simulink model "test"  (R2018b)
settings: Solver=VariableStepAuto  StartTime=0.0  StopTime=10.0  RelTol=1e-3
values from neighbouring files (symbols this model uses):
  A_bike = [0 g/h_real ; 1 0]    [configuration.m]
  A_bike_dis_prediction = A_bike_dis^d_delay    [configuration.m]    (also in prediction_smith.m)
  B_bike = [1 ; 0]    [configuration.m]
  B_bike_dis_prediction = vec_powers_AB    [configuration.m]    (also in prediction_smith.m)
  C1_bike = a_real/(b_real*h_real)    (= 0.392543973584)    [configuration.m]
  C2_bike = 1/(b_real*h_real)    (= 1.15454109878)    [configuration.m]
  C_ini = [C1_bike*input_velocity C2_bike*input_velocity^2]    [configuration.m]
  D = zeros(3,1)    [configuration_pidTuning.m]
  d_delay = delay_tf_steering/Ts    (= 0)    [configuration.m]    (also in prediction_smith.m = 3)
  D_steering_position = 0.0    (= 0)    [configuration.m]
  delay_tf_steering = 0    [configuration.m]
  den_tf_steering = [1 245.9 0]    [configuration.m]
  den_tf_steering_dis = [den_tf_steering_dis 0] - [0 den_tf_steering_dis]    [configuration.m]
  I_steering_position = 1    [configuration.m]    (also in simulate_bike.m = 30)
  initial_states = [deg2rad(-2) deg2rad(0) deg2rad(0)]    [configuration.m]    (also in configuration_pidTuning.m)
  input_velocity = 4    [configuration.m]    (also in configuration_pidTuning.m = 3)
  K_feedforward_steering = 0    [configuration.m]
  K_fullbike = 1    [configuration.m]
  lqr_gains = zeros(length(velocity_lqr),1+size(A_bike,1))    [lqr_design.m]
  max_steering_motor_speed = 0.9    [configuration.m]    (also in configuration_pidTuning.m = 7.5)
  min_steering_motor_speed = -0.9    [configuration.m]    (also in configuration_pidTuning.m = -7.5)
  num_tf_steering = [253.4]    [configuration.m]
  num_tf_steering_dis = [num_tf_steering_dis 0]    [configuration.m]
  P_steering_position = 10    [configuration.m]    (also in simulate_bike.m = 30)
  smith_fullbike = 1    [configuration.m]
  smith_steering = 0    [configuration.m]
  Ts = 0.01    [configuration.m]    (also in configuration_pidTuning.m = 0.04)
  velocity_lqr = [input_velocity - 0.1 , input_velocity , input_velocity + 0.1]    [lqr_design.m]
undefined symbols (not defined in the file or in its folder): a_steering_filter, b_steering_filter
libraries: simulink x3
settings Model: Creator=maximef  LastModifiedBy=maximef

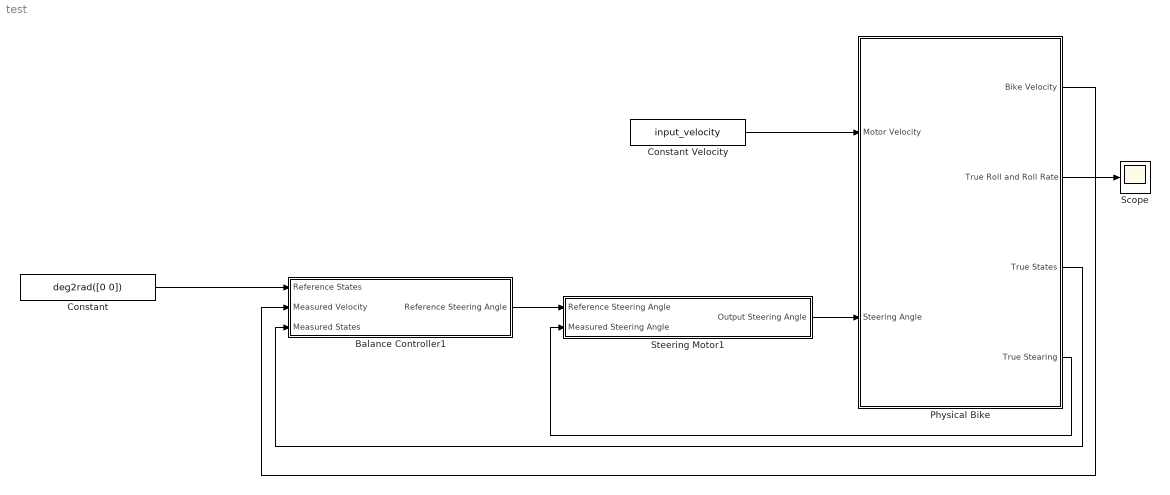
== system test ==
  Balance Controller1 : Subsystem  SystemSampleTime=Ts
  Constant : Constant  Value=deg2rad([0 0])
  Constant Velocity : Constant  Value=input_velocity
  Physical Bike : Subsystem
  Scope : Scope
  Steering Motor1 : Subsystem
  wires:
  Balance Controller1/1(Reference Steering Angle) -> Steering Motor1/1(Reference Steering Angle)
  Steering Motor1/1(Output Steering Angle) -> Physical Bike/2(Steering Angle)
  Physical Bike/3(True States) -> Balance Controller1/3(Measured States)
  Physical Bike/1(Bike Velocity) -> Balance Controller1/2(Measured Velocity)
  Physical Bike/2(True Roll and Roll Rate) -> Scope/1
  Physical Bike/4(True Stearing) -> Steering Motor1/2(Measured Steering Angle)
  Constant Velocity/1 -> Physical Bike/1(Motor Velocity)
  Constant/1 -> Balance Controller1/1(Reference States)

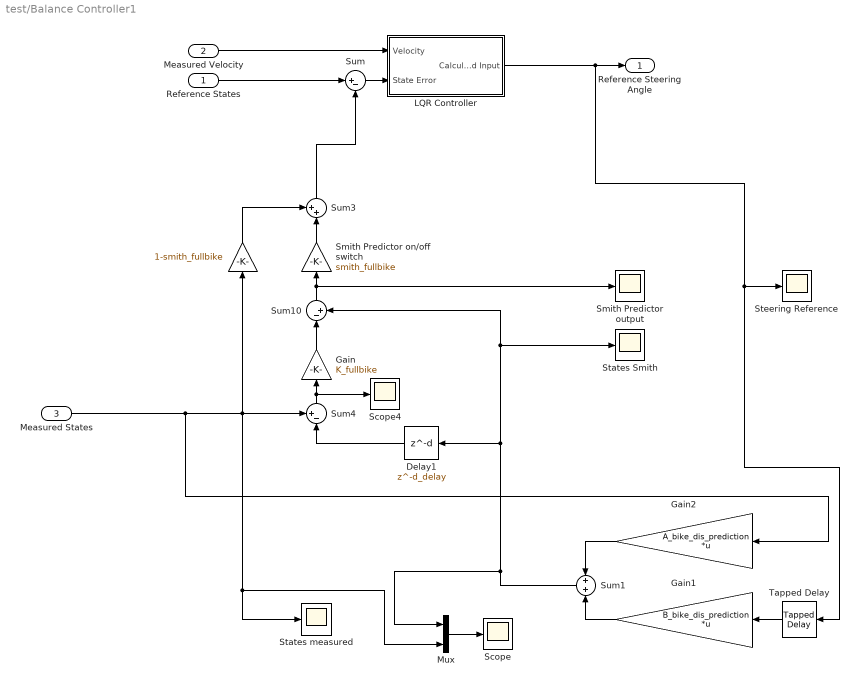
== system test/Balance Controller1 ==
  Reference States : Inport
  Measured Velocity : Inport  Port=2
  Measured States : Inport  Port=3
  " " : Gain  Gain=1-smith_fullbike
  Delay1 : Delay  DelayLength=d_delay  SampleTime=Ts
  Gain : Gain  Gain=K_fullbike
  Gain1 : Gain  Gain=B_bike_dis_prediction  Multiplication=Matrix(K*u)
  Gain2 : Gain  Gain=A_bike_dis_prediction  Multiplication=Matrix(K*u)
  LQR Controller : Subsystem  TreatAsAtomicUnit=on  SystemSampleTime=Ts
  Mux : Mux  Inputs=2
  Scope : Scope
  Scope4 : Scope
  Smith Predictor on/off switch : Gain  Gain=smith_fullbike
  Smith Predictor output : Scope
  States Smith : Scope
  States measured : Scope
  Steering Reference : Scope
  Sum : Sum  Inputs=|+-
  Sum1 : Sum
  Sum10 : Sum  Inputs=|-+
  Sum3 : Sum  Inputs=++|
  Sum4 : Sum  Inputs=+-|
  Tapped Delay : simulink/Discrete/Tapped Delay  vinit=0.0  samptime=Ts  NumDelays=d_delay  DelayOrder=Oldest  includeCurrent=off
  Reference Steering Angle : Outport
  wires:
  Sum/1 -> LQR Controller/2(State Error)
  " "/1 -> Sum3/1
  Sum3/1 -> Sum/2
  Gain/1 -> Sum10/1
  Delay1/1 -> Sum4/2
  Smith Predictor on/off switch/1 -> Sum3/2
  Sum10/1 -> Smith Predictor output/1, Smith Predictor on/off switch/1
  Sum4/1 -> Scope4/1, Gain/1
  LQR Controller/1(Calculated Input) -> Tapped Delay/1, Steering Reference/1, Reference Steering Angle/1
  Measured Velocity/1 -> LQR Controller/1(Velocity)
  Gain1/1 -> Sum1/2
  Tapped Delay/1 -> Gain1/1
  Gain2/1 -> Sum1/1
  Sum1/1 -> Sum10/2, States Smith/1, Delay1/1, Mux/1
  Mux/1 -> Scope/1
  Measured States/1 -> Gain2/1, " "/1, States measured/1, Mux/2, Sum4/1
  Reference States/1 -> Sum/1

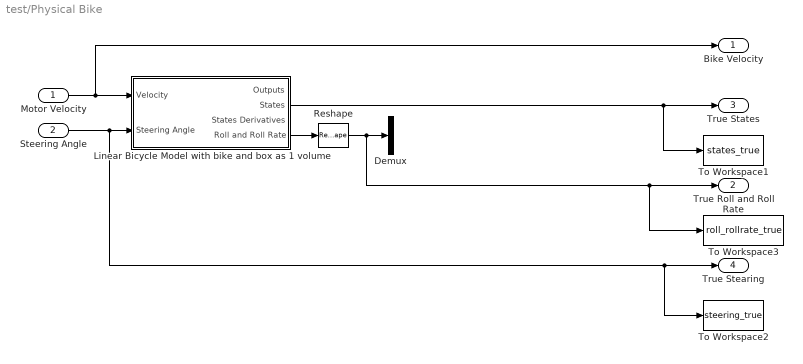
== system test/Physical Bike ==
  Motor Velocity : Inport
  Steering Angle : Inport  Port=2
  Demux : Demux  Outputs=2
  Linear Bicycle Model with bike and box as 1 volume : Subsystem
  Reshape : Reshape
  To Workspace1 : ToWorkspace  VariableName=states_true  SaveFormat=Timeseries  SampleTime=-1
  To Workspace2 : ToWorkspace  VariableName=steering_true  SaveFormat=Timeseries  SampleTime=-1
  To Workspace3 : ToWorkspace  VariableName=roll_rollrate_true  SaveFormat=Timeseries  SampleTime=-1
  Bike Velocity : Outport
  True Roll and Roll Rate : Outport  Port=2
  True States : Outport  Port=3
  True Stearing : Outport  Port=4
  wires:
  Steering Angle/1 -> To Workspace2/1, True Stearing/1, Linear Bicycle Model with bike and box as 1 volume/2(Steering Angle)
  Motor Velocity/1 -> Bike Velocity/1, Linear Bicycle Model with bike and box as 1 volume/1(Velocity)
  Linear Bicycle Model with bike and box as 1 volume/2(States) -> To Workspace1/1, True States/1
  Linear Bicycle Model with bike and box as 1 volume/4(Roll and Roll Rate) -> Reshape/1
  Reshape/1 -> To Workspace3/1, True Roll and Roll Rate/1, Demux/1

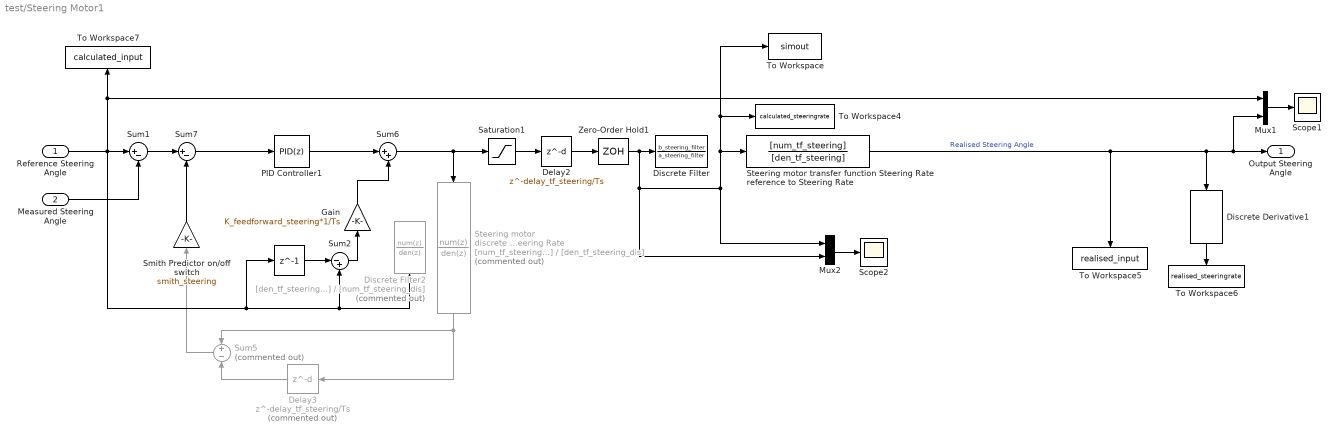
== system test/Steering Motor1 ==
  Reference Steering Angle : Inport
  Measured Steering Angle : Inport  Port=2
  " " : Delay  DelayLength=1  SampleTime=Ts
  Delay2 : Delay  DelayLength=delay_tf_steering/Ts  SampleTime=Ts
  Delay3 : Delay  Commented=on  DelayLength=delay_tf_steering/Ts  SampleTime=Ts
  Discrete Derivative1 : simulink/Discrete/Discrete Derivative  gainval=1.0  ICPrevScaledInput=0.0  OutMin=[]  OutMax=[]  OutDataType=fixdt(1, 16)  OutScaling=2^-10  DoSatur=off
  Discrete Filter : DiscreteFilter  Numerator=b_steering_filter  Denominator=a_steering_filter  SampleTime=Ts
  Discrete Filter2 : DiscreteFilter  Commented=on  Numerator=[den_tf_steering_dis]  Denominator=[num_tf_steering_dis]
  Gain : Gain  Gain=K_feedforward_steering*1/Ts
  Mux1 : Mux  Inputs=2
  Mux2 : Mux  Inputs=2
  PID Controller1 : simulink/Continuous/PID Controller  Controller=PID  Form=Parallel  TimeDomain=Discrete-time  SampleTime=Ts  IntegratorMethod=Forward Euler  FilterMethod=Forward Euler  ControllerParametersSource=internal  P=P_steering_position  I=I_steering_position  D=D_steering_position  UseFilter=off  N=1  TunerSelectOption=Transfer Function Based (PID Tuner App)  InitialConditionSource=internal  InitialConditionForIntegrator=0  InitialConditionForFilter=0  DifferentiatorICPrevScaledInput=0  ExternalReset=none  TrackingMode=off  Kt=1  LimitOutput=off  UpperSaturationLimit=inf  LowerSaturationLimit=-inf  LinearizeAsGain=on  AntiWindupMode=none  Kb=1  POutMin=[]  POutMax=[]  IOutMin=[]  IOutMax=[]  DOutMin=[]  DOutMax=[]  NOutMin=[]  NOutMax=[]  SumOutMin=[]  SumOutMax=[]  SaturationOutMin=[]  SaturationOutMax=[]  PParamMin=[]  PParamMax=[]  IParamMin=[]  IParamMax=[]  DParamMin=[]  DParamMax=[]  NParamMin=[]  NParamMax=[]  KbParamMin=[]  KbParamMax=[]  KtParamMin=[]  KtParamMax=[]  KbOutMin=[]  KbOutMax=[]  KtOutMin=[]  KtOutMax=[]  IntegratorOutMin=[]  IntegratorOutMax=[]  FilterOutMin=[]  FilterOutMax=[]  SumI1OutMin=[]  SumI1OutMax=[]  SumI2OutMin=[]  SumI2OutMax=[]  SumI3OutMin=[]  SumI3OutMax=[]  SumI4OutMin=[]  SumI4OutMax=[]  SumDOutMin=[]  SumDOutMax=[]  DifferentiatorOutMin=[]  DifferentiatorOutMax=[]  FilterDiffOutCoefMin=[]  FilterDiffOutCoefMax=[]  ReciprocalOutMin=[]  ReciprocalOutMax=[]  SumDenOutMin=[]  SumDenOutMax=[]  SumNumOutMin=[]  SumNumOutMax=[]  DivideOutMin=[]  DivideOutMax=[]  IntegratorContinuousStateAttributes=''  IntegratorStateMustResolveToSignalObject=off  IntegratorRTWStateStorageClass=Auto  FilterContinuousStateAttributes=''  FilterStateMustResolveToSignalObject=off  FilterRTWStateStorageClass=Auto  ParallelPVariant=InternalParameters  IdealPVariant=Disabled  IVariant=InternalParameters  DVariant=InternalParameters  IntegratorVariant=Discrete  SatVariant=Disabled  AWVariant=Passthrough  PCopyVariant=Disabled  TRVariant=Disabled  FdbkBlocksVariant=Forward  IdealPFdbkVariant=Disabled  SatFdbkVariant=Disabled  DerivativeFilterVariant=Differentiator  NVariant=Passthrough  NCopyVariant=Disabled_SignalSpec  FilterICVariant=InternalICsDifferentiator  IntegratorICVariant=InternalICs  ExternalResetVariant=Disabled  TRSumVariant=Passthrough  SumFdbkVariant=Disabled  SumVariant=Sum_PID
  Saturation1 : Saturate  UpperLimit=max_steering_motor_speed  LowerLimit=min_steering_motor_speed
  Scope1 : Scope
  Scope2 : Scope
  Smith Predictor on/off switch : Gain  Gain=smith_steering
  Steering motor discrete transfer function Steering Rate reference to Steering Rate : DiscreteTransferFcn  Commented=on  Numerator=[num_tf_steering_dis]  Denominator=[den_tf_steering_dis]  SampleTime=Ts
  Steering motor transfer function Steering Rate reference to Steering Rate : TransferFcn  Numerator=[num_tf_steering]  Denominator=[den_tf_steering]
  Sum1 : Sum  Inputs=|+-
  Sum2 : Sum  Inputs=|-+
  Sum5 : Sum  Commented=on  Inputs=+-
  Sum6 : Sum  Inputs=|++
  Sum7 : Sum  Inputs=|+-
  To Workspace : ToWorkspace  VariableName=simout  SaveFormat=Timeseries  SampleTime=-1
  To Workspace4 : ToWorkspace  VariableName=calculated_steeringrate  SaveFormat=Timeseries  SampleTime=-1
  To Workspace5 : ToWorkspace  VariableName=realised_input  SaveFormat=Timeseries  SampleTime=-1
  To Workspace6 : ToWorkspace  VariableName=realised_steeringrate  SaveFormat=Timeseries  SampleTime=-1
  To Workspace7 : ToWorkspace  VariableName=calculated_input  SaveFormat=Timeseries  SampleTime=Ts
  Zero-Order Hold1 : ZeroOrderHold  SampleTime=Ts
  Output Steering Angle : Outport
  wires:
  Saturation1/1 -> Delay2/1
  Steering motor discrete transfer function Steering Rate reference to Steering Rate/1 -> Delay3/1, Sum5/1
  Sum5/1 -> Smith Predictor on/off switch/1
  Delay3/1 -> Sum5/2
  Mux1/1 -> Scope1/1
  Sum6/1 -> Saturation1/1, Steering motor discrete transfer function Steering Rate reference to Steering Rate/1
  Sum1/1 -> Sum7/1
  Smith Predictor on/off switch/1 -> Sum7/2
  Delay2/1 -> Zero-Order Hold1/1
  Steering motor transfer function Steering Rate reference to Steering Rate/1 -> Discrete Derivative1/1, Mux1/2, Output Steering Angle/1, To Workspace5/1  "Realised Steering Angle"
  Reference Steering Angle/1 -> Discrete Filter2/1, Sum2/2, " "/1, Sum1/1, Mux1/1, To Workspace7/1
  Discrete Derivative1/1 -> To Workspace6/1
  Measured Steering Angle/1 -> Sum1/2
  " "/1 -> Sum2/1
  Sum2/1 -> Gain/1
  Gain/1 -> Sum6/2
  Sum7/1 -> PID Controller1/1
  PID Controller1/1 -> Sum6/1
  Mux2/1 -> Scope2/1
  Zero-Order Hold1/1 -> Steering motor transfer function Steering Rate reference to Steering Rate/1, To Workspace/1, To Workspace4/1, Mux2/1, Mux2/2, Discrete Filter/1

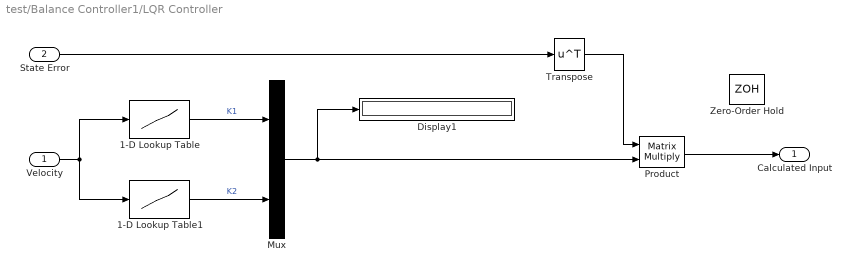
== system test/Balance Controller1/LQR Controller ==
  Velocity : Inport
  State Error : Inport  Port=2
  1-D Lookup Table : Lookup_n-D  NumberOfTableDimensions=1  BreakpointsForDimension1=velocity_lqr  BreakpointsForDimension2=velocity_lqr  BreakpointsForDimension3=velocity_lqr  BreakpointsForDimension4=velocity_lqr  Table=lqr_gains(:,2)  InternalRulePriority=Speed  RndMeth=Simplest  InputSameDT=on
  1-D Lookup Table1 : Lookup_n-D  NumberOfTableDimensions=1  BreakpointsForDimension1=velocity_lqr  BreakpointsForDimension2=velocity_lqr  BreakpointsForDimension3=velocity_lqr  BreakpointsForDimension4=velocity_lqr  Table=lqr_gains(:,3)  InternalRulePriority=Speed  RndMeth=Simplest  InputSameDT=on
  Display1 : Display
  Mux : Mux  Inputs=2
  Product : Product  Multiplication=Matrix(*)
  Transpose : Math  Operator=transpose  SaturateOnIntegerOverflow=on
  Zero-Order Hold : ZeroOrderHold  SampleTime=Ts
  Calculated Input : Outport
  wires:
  1-D Lookup Table/1 -> Mux/1  "K1"
  1-D Lookup Table1/1 -> Mux/2  "K2"
  Velocity/1 -> 1-D Lookup Table1/1, 1-D Lookup Table/1
  Mux/1 -> Product/2, Display1/1
  Transpose/1 -> Product/1
  Product/1 -> Calculated Input/1
  State Error/1 -> Transpose/1

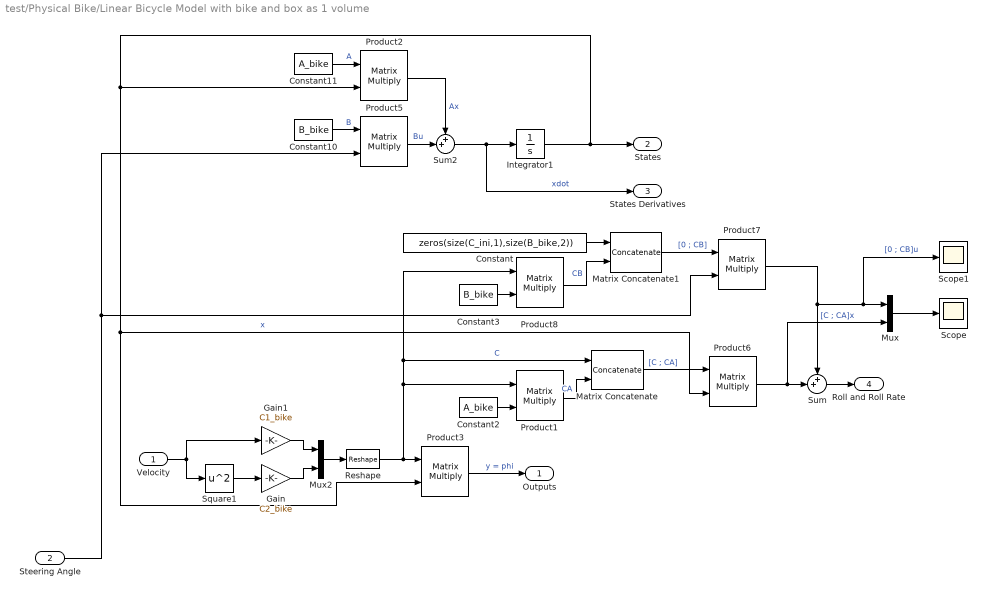
== system test/Physical Bike/Linear Bicycle Model with bike and box as 1 volume ==
  Velocity : Inport
  Steering Angle : Inport  Port=2
  Constant : Constant  Value=zeros(size(C_ini,1),size(B_bike,2))
  Constant10 : Constant  Value=B_bike
  Constant11 : Constant  Value=A_bike
  Constant2 : Constant  Value=A_bike
  Constant3 : Constant  Value=B_bike
  Gain : Gain  Gain=C2_bike
  Gain1 : Gain  Gain=C1_bike
  Integrator1 : Integrator  InitialCondition=[C_ini ; C_ini*A_bike]\[initial_states(1) ; initial_states(3)]
  Matrix Concatenate : Concatenate  Mode=Multidimensional array
  Matrix Concatenate1 : Concatenate  Mode=Multidimensional array
  Mux : Mux  Inputs=2
  Mux2 : Mux  Inputs=2
  Product{1..3,5..8} (7 alike) : Product  SCDEnableBlockLinearizationSpecification=on  Multiplication=Matrix(*)
  Reshape : Reshape  OutputDimensionality=Row vector (2-D)
  Scope : Scope
  Scope1 : Scope
  Square1 : Math  Operator=square  SaturateOnIntegerOverflow=on
  Sum : Sum  Inputs=++|
  Sum2 : Sum  Inputs=++|
  Outputs : Outport
  States : Outport  Port=2
  States Derivatives : Outport  Port=3
  Roll and Roll Rate : Outport  Port=4
  wires:
  Integrator1/1 -> Product2/2, Product6/2, Product3/2, States/1  "x"
  Product3/1 -> Outputs/1  "y = phi"
  Steering Angle/1 -> Product5/2, Product7/2
  Product2/1 -> Sum2/1  "Ax"
  Mux2/1 -> Reshape/1
  Product5/1 -> Sum2/2  "Bu"
  Sum2/1 -> Integrator1/1, States Derivatives/1  "xdot"
  Constant11/1 -> Product2/1  "A"
  Constant10/1 -> Product5/1  "B"
  Velocity/1 -> Gain1/1, Square1/1
  Square1/1 -> Gain/1
  Reshape/1 -> Product3/1, Product8/1, Matrix Concatenate/1, Product1/1  "C"
  Gain/1 -> Mux2/2
  Gain1/1 -> Mux2/1
  Sum/1 -> Roll and Roll Rate/1
  Constant2/1 -> Product1/2
  Product1/1 -> Matrix Concatenate/2  "CA"
  Matrix Concatenate/1 -> Product6/1  "[C ; CA]"
  Product6/1 -> Mux/2, Sum/2  "[C ; CA]x"
  Product7/1 -> Scope1/1, Mux/1, Sum/1  "[0 ; CB]u"
  Matrix Concatenate1/1 -> Product7/1  "[0 ; CB]"
  Product8/1 -> Matrix Concatenate1/2  "CB"
  Constant3/1 -> Product8/2
  Constant/1 -> Matrix Concatenate1/1
  Mux/1 -> Scope/1
